simulink model "controler_sim"  (R2020a)
settings: Solver=VariableStepAuto  StartTime=0.0  StopTime=300  RelTol=1e-3
settings Model: Creator=Alexander Grebien  LastModifiedBy=Alexander Grebien

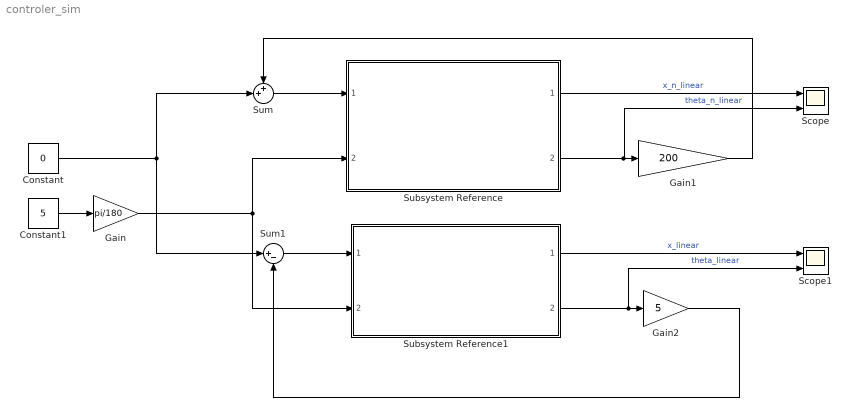
== system controler_sim ==
  Constant : Constant  Value=0
  Constant1 : Constant  Value=5
  Gain : Gain  Gain=pi/180
  Gain1 : Gain  Gain=200
  Gain2 : Gain  Gain=5
  Scope : Scope  NumInputPorts=2
  Scope1 : Scope  NumInputPorts=2
  Subsystem Reference : Subsystem  ReferencedSubsystem=non_linear_model
  Subsystem Reference1 : Subsystem  ReferencedSubsystem=linearized_model
  Sum : Sum  Inputs=++|
  Sum1 : Sum  Inputs=|+-
  wires:
  Subsystem Reference1/2 -> Scope1/2, Gain2/1  "theta_linear"
  Sum1/1 -> Subsystem Reference1/1
  Subsystem Reference/2 -> Scope/2, Gain1/1  "theta_n_linear"
  Sum/1 -> Subsystem Reference/1
  Subsystem Reference/1 -> Scope/1  "x_n_linear"
  Subsystem Reference1/1 -> Scope1/1  "x_linear"
  Constant/1 -> Sum1/1, Sum/2
  Constant1/1 -> Gain/1
  Gain/1 -> Subsystem Reference/2, Subsystem Reference1/2
  Gain1/1 -> Sum/1
  Gain2/1 -> Sum1/2
